simulink model "conv_AM_envelope"  (R2021a)
settings: Solver=VariableStepAuto  StartTime=0.0  StopTime=10.0  RelTol=1e-3
libraries: dsparch4 x1, dspsigops x1
settings Model: Creator=Fatiha  LastModifiedBy=Fatiha

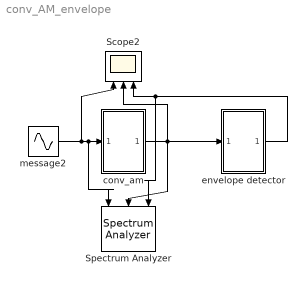
== system conv_AM_envelope ==
  Scope2 : Scope  NumInputPorts=3
  Spectrum Analyzer : SpectrumAnalyzer  NumInputPorts=3
  conv_am : Subsystem
  envelope detector : Subsystem
  message2 : Sin  Frequency=2*pi*50  Phase=pi/2  SampleTime=0.00001
  wires:
  conv_am/1(Out1) -> envelope detector/1(In1), Spectrum Analyzer/2, Scope2/2
  message2/1 -> Spectrum Analyzer/1, conv_am/1(In1), Scope2/1
  envelope detector/1(Out1) -> Scope2/3, Spectrum Analyzer/3

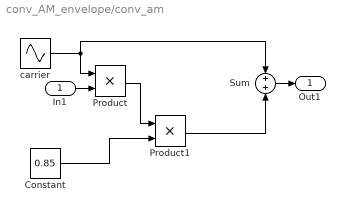
== system conv_AM_envelope/conv_am ==
  In1 : Inport
  Constant : Constant  Value=0.85
  Product : Product
  Product1 : Product
  Sum : Sum  Inputs=+|+
  carrier : Sin  Frequency=2*pi*500  Phase=pi/2  SampleTime=0.00001
  Out1 : Outport
  wires:
  Product1/1 -> Sum/2
  In1/1 -> Product/2
  carrier/1 -> Product/1, Sum/1
  Constant/1 -> Product1/2
  Product/1 -> Product1/1
  Sum/1 -> Out1/1

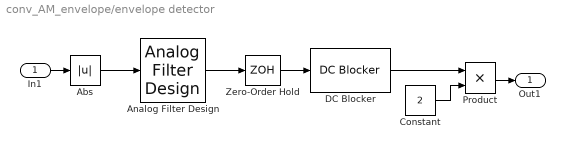
== system conv_AM_envelope/envelope detector ==
  In1 : Inport
  Abs : Abs
  Analog Filter Design : dsparch4/Analog Filter Design  method=Butterworth  filttype=Lowpass  N=8  Wlo=2*pi*0.5e3  Whi=80  Rp=2  Rs=40
  Constant : Constant  Value=2
  DC Blocker : dspsigops/DC Blocker  Algorithm=IIR  NormalizedBandwidth=0.001  Length=8  Order=6  SimulateUsing=Code generation
      settings: SourceProductBaseCode=DS
  Product : Product
  Zero-Order Hold : ZeroOrderHold  SampleTime=-1
  Out1 : Outport
  wires:
  DC Blocker/1 -> Product/1
  Product/1 -> Out1/1
  In1/1 -> Abs/1
  Constant/1 -> Product/2
  Analog Filter Design/1 -> Zero-Order Hold/1
  Zero-Order Hold/1 -> DC Blocker/1
  Abs/1 -> Analog Filter Design/1
